simulink model "cruise_control_statemachine"  (R2018a)
settings: Solver=FixedStepAuto  StartTime=0.0  StopTime=inf  RelTol=1e-3  EnableMultiTasking=on
undefined symbols (not defined in the file): Angular, Linear
libraries: robotlib x2
settings Model: Creator=ece446  LastModifiedBy=ivory
settings OptimizationCC: LifeSpan=Inf  MaxStackSize=64
settings DebuggingCC: SFUnexpectedBacktrackingDiag=warning  SFNoUnconditionalDefaultTransitionDiag=warning  SFExecutionAtInitializationDiag=none
settings HardwareCC: ProdBitPerPointer=32  ProdBitPerSizeT=32  ProdBitPerPtrDiffT=32  ProdLargestAtomicFloat=None  ProdIntDivRoundTo=Undefined  ProdEndianess=Unspecified  ProdWordSize=32  ProdHWDeviceType=Generic->Unspecified (assume 32-bit Generic)  UseEmbeddedCoderFeatures=off
settings RTWCC: SystemTargetFile=ert.tlc  HardwareBoard=Robot Operating System (ROS)  TLCOptions=-aInlineSetEventsForThisBaseRateFcn=TLC_FALSE -aSuppressMultiTaskScheduler=TLC_FALSE -aRateBasedStepFcn=0  TemplateMakefile=ert_default_tmf  GenerateReport=on  Toolchain=Catkin  LaunchReport=on  TargetLang=C++
settings CodeAppCC: ForceParamTrailComments=on  OperatorAnnotations=on  StateflowObjectComments=on  MATLABSourceComments=on
settings ERTTargetCC: MultiwordLength=2048  ERTCustomFileBanners=off  SupportContinuousTime=on  SupportNonInlinedSFcns=on  RemoveResetFunc=off  ModelStepFunctionPrototypeControlCompliant=off
settings ConfigComp: CovMetricSettings=dw  CovHtmlReporting=on  CovSaveCumulativeToWorkspaceVar=on  CovSaveSingleToWorkspaceVar=on  CovExternalEMLEnable=off

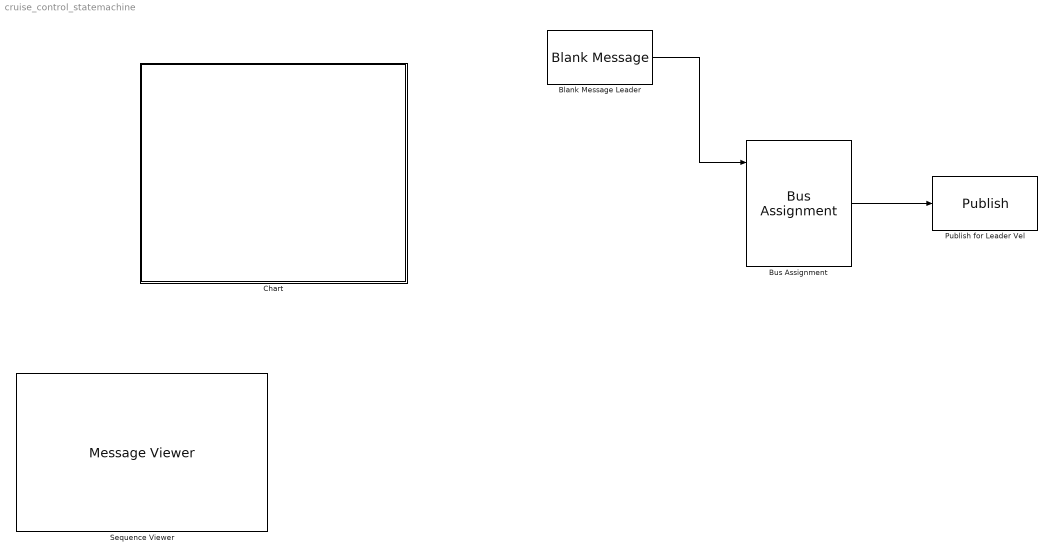
== system cruise_control_statemachine ==
  Blank Message Leader : robotlib/Blank Message  SourceLibraryInfo=This block requires Robotics System Toolbox  messageType=geometry_msgs/Twist  SampleTime=inf
      settings: SourceProductBaseCode=RO
  Bus Assignment : BusAssignment  AssignedSignals=Linear.X,Angular.Z
  Chart : Stateflow chart  TreatAsAtomicUnit=on
  Publish for Leader Vel : robotlib/Publish  SourceLibraryInfo=This block requires Robotics System Toolbox  topicSource=Specify your own  topic=cmd_vel  messageType=geometry_msgs/Twist  messageQueueLength=1
      settings: SourceProductBaseCode=RO
  Sequence Viewer : MessageViewer
  wires:
  Blank Message Leader/1 -> Bus Assignment/1
  Bus Assignment/1 -> Publish for Leader Vel/1

== stateflow chart cruise_control_statemachine/Chart ==
  state Stay
    entry: entryState = exitState; u2 = v; t0 = getROStime();
    during: deltaT = getROStime() - t0;
    exit: exitState = entryState + 1;
  state DecelerateTo35
    entry: entryState = exitState; t0 = getROStime();
    during: v = getNewV(u2, delpha, t0);
    exit: exitState = entryState + 1;
  state AccelerateTo55_init
    entry: entryState = 0; t0 = getROStime();
    during: v = getNewV(u, alpha, t0)
    exit:  exitState = entryState + 1;
  state zero
    entry: v = 0;
    during:v = 0;
  note: STATE 1
  note: STATE 2, 4, 6, 8, 10
  note: STATE 3
  state DecelerateTo45
    entry: entryState = exitState; t0 = getROStime();
    during: v = getNewV(u2, delpha, t0);
    exit: exitState = entryState + 1;
  state DecelerateTo46
    entry: entryState = exitState; t0 = getROStime();
    during: v = getNewV(u2, delpha, t0);
    exit: exitState = entryState + 1;
  state AccelerateTo55
    entry: t0 = getROStime(); stateIndex = 1
    during: v = getNewV(u2, alpha, t0)
  note: STATE 5
  note: STATE 7
  note: [v >= 35 && exitState = 5]
  (default) -> AccelerateTo55_init
  DecelerateTo35 -> DecelerateTo35 [order 2] : [v > 35]
  Stay -> DecelerateTo35 [order 2] : [deltaT > 60 && exitState == 2]
  AccelerateTo55_init -> Stay [order 2] : [v>=55 ]
  Stay -> Stay [order 1] : [deltaT <= 60]
  DecelerateTo35 -> Stay [order 1] : [v <= 35 && exitState = 3]
  Stay -> DecelerateTo45 [order 4] : [deltaT > 60 && exitState == 6]
  AccelerateTo55_init -> AccelerateTo55_init [order 1] : [v < 55]
  Stay -> DecelerateTo46 [order 5] : [deltaT > 60 && exitState== 10]
  AccelerateTo55 -> Stay [order 1] : [v >= 55 && (exitState == 5 || exitState == 9)]
  Stay -> AccelerateTo55 [order 3] : [deltaT > 60 && (exitState == 4 || exitState == 8)]
  DecelerateTo45 -> Stay [order 2] : [v <= 45 && exitState = 7]
  DecelerateTo46 -> zero [order 2] : [v <=0]
  DecelerateTo45 -> DecelerateTo45 [order 1] : [v > 45]
  AccelerateTo55 -> AccelerateTo55 [order 2] : [deltaT <=60]
  DecelerateTo46 -> DecelerateTo46 [order 1] : [v > 0]
  data: init_velocity function_input; acceleration function_input; initial_time function_input; v function_output; t function_output
  function v = getNewV(init_velocity, acceleration, initial_time):
    | function v = getNewV(init_velocity, acceleration, initial_time)
    | 
    | v = init_velocity + acceleration*(rostime('now') - initial_time);
    | 
    | end
  function t = getROStime:
    | function t = getROStime()
    |     t = rostime('now');
    | end
